simulink model "scars_example_backup"  (R2019b)
settings: Solver=ode14x  StartTime=0.0  StopTime=400  FixedStep=dT  RelTol=1e-3
libraries: scars_library x9
settings Model: Creator=asmialek  LastModifiedBy=asmialek
settings DataIOCC: ReturnWorkspaceOutputsName=scars_out

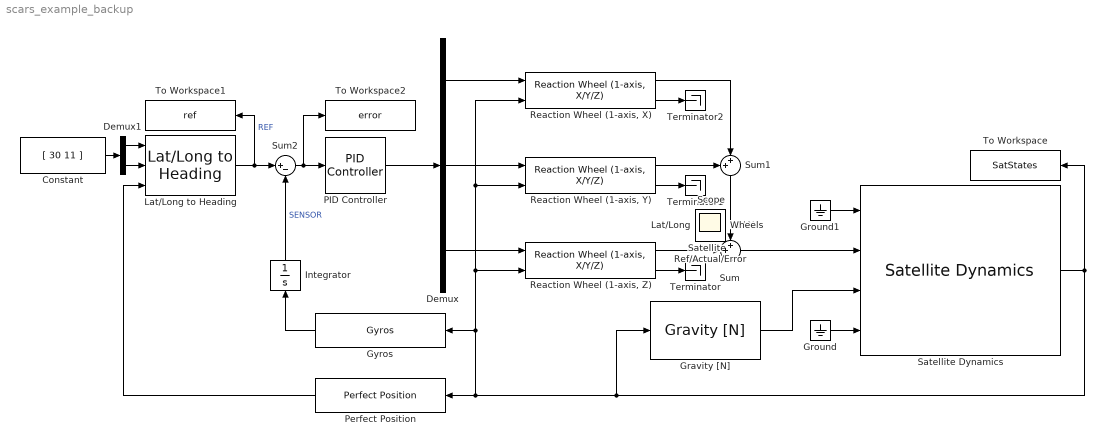
== system scars_example_backup ==
  Constant : Constant  Value=[ 30 11 ]
  Demux : Demux  Outputs=3
  Demux1 : Demux  Outputs=2
  Gravity [N] : scars_library/Environment/Gravity [N]  mass=1
  Ground : Ground
  Ground1 : Ground
  Gyros : scars_library/Sensors/Gyros  g_wn=14500  g_zeta=sqrt(2)/2  g_freq=10  g_bias=0  g_power=(2*pi*0.04/360)^2  g_max=deg2rad(75)  g_min=-deg2rad(75)
  Integrator : Integrator  InitialCondition=deg2rad([0 0 0])
  Lat/Long to Heading : scars_library/ Control Algorithms /Lat//Long to Heading  SystemSampleTime=-1  Latency=0  AutoFrameSizeCalculation=off
  PID Controller : scars_library/ Control Algorithms /PID Controller  Kp=1  Ki=1e-4  Kd=100  pid_sat_max=inf  pid_sat_min=-inf  pid_dz_max=0  pid_dz_min=0
  Perfect Position : scars_library/Sensors/Perfect Position  SystemSampleTime=-1  Latency=0  AutoFrameSizeCalculation=off
  "Reaction Wheel (1-axis, X)" : scars_library/Actuators/Reaction Wheel (1-axis, X//Y//Z)  axis_switch=X  N=(1.5e-3)/0.5  R=12  J=300e-3  c=0.0001  vel_max=6000*2*pi/60  torq_max=1.5e-3  i_max=0.5  rw_power=0  rw_freq=0.1
  "Reaction Wheel (1-axis, Y)" : scars_library/Actuators/Reaction Wheel (1-axis, X//Y//Z)  axis_switch=Y  N=(1.5e-3)/0.5  R=12  J=300e-3  c=0.0001  vel_max=6000*2*pi/60  torq_max=1.5e-3  i_max=0.5  rw_power=0  rw_freq=0.1
  "Reaction Wheel (1-axis, Z)" : scars_library/Actuators/Reaction Wheel (1-axis, X//Y//Z)  axis_switch=Z  N=(1.5e-3)/0.5  R=12  J=300e-3  c=0.0001  vel_max=6000*2*pi/60  torq_max=1.5e-3  i_max=0.5  rw_power=0  rw_freq=0.1
  Satellite Dynamics : scars_library/Advanced/Satellite Dynamics  Parameter4=LLA Position & NED Velocity, Rotation  epoch=2451545  mass=1  a=6356e3+400e3  e=0  incl=10  RA=209.369  w=0  TA=96  initEuler=[0 0 0]  initEulerRates=[0.01 0.02 0.005]  TA_copy=0  TA_copy_copy=400e3  TA_copy_copy_copy=[10 25]  TA_copy_copy_copy_copy=[1332.41761449570 7062.27056473502 -0.000303983477717348]  initEuler_copy=[0 0 0]  initEulerRates_copy=[0.01 0.02 0.005]  mask(Sattellite Dynamics){}
  Sum : Sum  Inputs=++|
  Sum1 : Sum  Inputs=++|
  Sum2 : Sum  Inputs=|+-
  Terminator : Terminator
  Terminator1 : Terminator
  Terminator2 : Terminator
  To Workspace : ToWorkspace  VariableName=SatStates  SaveFormat=Timeseries  SampleTime=-1
  To Workspace1 : ToWorkspace  VariableName=ref  SaveFormat=Timeseries  SampleTime=-1
  To Workspace2 : ToWorkspace  VariableName=error  SaveFormat=Timeseries  SampleTime=-1
  Lat/Long : Scope
  RW Y : Scope
  Ref/Actual/Error : Scope
  Satellite : Scope
  Scope : Scope
  Wheels : Scope
  wires:
  Ground/1 -> Satellite Dynamics/4
  Gravity [N]/1 -> Satellite Dynamics/3
  Satellite Dynamics/1 -> Perfect Position/1, Gyros/1, "Reaction Wheel (1-axis, X)"/2, "Reaction Wheel (1-axis, Y)"/2, "Reaction Wheel (1-axis, Z)"/2, Gravity [N]/1, To Workspace/1
  Ground1/1 -> Satellite Dynamics/1
  "Reaction Wheel (1-axis, Z)"/1 -> Sum/2
  "Reaction Wheel (1-axis, Z)"/2 -> Terminator/1
  "Reaction Wheel (1-axis, Y)"/2 -> Terminator1/1
  "Reaction Wheel (1-axis, X)"/2 -> Terminator2/1
  Sum/1 -> Satellite Dynamics/2
  "Reaction Wheel (1-axis, Y)"/1 -> Sum1/1
  Sum1/1 -> Sum/1
  "Reaction Wheel (1-axis, X)"/1 -> Sum1/2
  Sum2/1 -> To Workspace2/1, PID Controller/1
  Lat/Long to Heading/1 -> To Workspace1/1, Sum2/1  "REF"
  Gyros/1 -> Integrator/1
  Demux/1 -> "Reaction Wheel (1-axis, X)"/1
  Demux/2 -> "Reaction Wheel (1-axis, Y)"/1
  Demux/3 -> "Reaction Wheel (1-axis, Z)"/1
  Demux1/1 -> Lat/Long to Heading/1
  Demux1/2 -> Lat/Long to Heading/2
  Constant/1 -> Demux1/1
  Perfect Position/1 -> Lat/Long to Heading/3
  Integrator/1 -> Sum2/2  "SENSOR"
  PID Controller/1 -> Demux/1
